simulink model "gm_Transformation_V12"  (R2018a)
settings: Solver=FixedStepDiscrete  StartTime=0.0  StopTime=10.0  RelTol=1e-3
InitFcn:
  | Ts_xadc = 0.1;
undefined symbols (not defined in the file or in its folder): T_25MHz, T_mech
libraries: hdlsllib x14, simulink x12, hdlmdlgenlib x5, simulink_need_slupdate x1
(part 3 of 4)

== matlab function gm_Transformation_V12/Trans_123_dq_fix_V3/dq_transformation ==
  data: a input; d output; b input; theta input; q output
% Author : Saeid Saeidi
% Modified: Sebastian Wendel
% EAL -TUM
% MATLAB Version : R2016a
function [d, q]= fcn(a,b, theta )
% Defining persistent variables
%In VHDL , persistent variables will appear as Signals
persistent i1
persistent i2
persistent i3
persistent i4
persistent i5
persistent i6
persistent i7
persistent i8
persistent i9
persistent i10
persistent i11
persistent i12
persistent i13
persistent i14
persistent i15
persistent i16
% %
persistent i1n
persistent i2n
persistent i3n
persistent i4n
persistent i5n
persistent i6n
persistent i7n
persistent i8n
persistent i9n
persistent i10n
persistent i11n
persistent i12n
persistent i13n
persistent i14n
persistent i15n
persistent i16n
% %
persistent a1
persistent a2
persistent a3
persistent a4
persistent a5
persistent a6
persistent a7
persistent a8
persistent a9
persistent a10
persistent a11
persistent a12
persistent a13
persistent a14
persistent a15
persistent a16
% %
persistent b1
persistent b2
persistent b3
persistent b4
persistent b5
persistent b6
persistent b7
persistent b8
persistent b9
persistent b10
persistent b11
persistent b12
persistent b13
persistent b14
persistent b15
persistent b16
% %
persistent beta1
persistent beta2
persistent beta3
persistent beta4
persistent beta5
persistent beta6
persistent beta7
persistent beta8
persistent beta9
persistent beta10
persistent beta11
persistent beta12
persistent beta13
persistent beta14
persistent beta15
% %
persistent a1n
persistent a2n
persistent a3n
persistent a4n
persistent a5n
persistent a6n
persistent a7n
persistent a8n
persistent a9n
persistent a10n
persistent a11n
persistent a12n
persistent a13n
persistent a14n
persistent a15n
persistent a16n
% %
persistent b1n
persistent b2n
persistent b3n
persistent b4n
persistent b5n
persistent b6n
persistent b7n
persistent b8n
persistent b9n
persistent b10n
persistent b11n
persistent b12n
persistent b13n
persistent b14n
persistent b15n
persistent b16n
% %
persistent beta1n
persistent beta2n
persistent beta3n
persistent beta4n
persistent beta5n
persistent beta6n
persistent beta7n
persistent beta8n
persistent beta9n
persistent beta10n
persistent beta11n
persistent beta12n
persistent beta13n
persistent beta14n
persistent beta15n
% %
% Initialization of Persistent Variables with the numeric type of the
% input variables "a" and "b"
% After generating VHDL this part will be located in the RESET
if isempty (a1)
a1 = fi (0, numerictype (a), hdlfimath );
a2 = fi (0, numerictype (a), hdlfimath );
a3 = fi (0, numerictype (a), hdlfimath );
a4 = fi (0, numerictype (a), hdlfimath );
a5 = fi (0, numerictype (a), hdlfimath );
a6 = fi (0, numerictype (a), hdlfimath );
a7 = fi (0, numerictype (a), hdlfimath );
a8 = fi (0, numerictype (a), hdlfimath );
a9 = fi (0, numerictype (a), hdlfimath );
a10 = fi (0, numerictype (a), hdlfimath );
a11 = fi (0, numerictype (a), hdlfimath );
a12 = fi (0, numerictype (a), hdlfimath );
a13 = fi (0, numerictype (a), hdlfimath );
a14 = fi (0, numerictype (a), hdlfimath );
a15 = fi (0, numerictype (a), hdlfimath );
a16 = fi (0, numerictype (a), hdlfimath );
% %
b1 = fi (0, numerictype (b), hdlfimath );
b2 = fi (0, numerictype (b), hdlfimath );
b3 = fi (0, numerictype (b), hdlfimath );
b4 = fi (0, numerictype (b), hdlfimath );
b5 = fi (0, numerictype (b), hdlfimath );
b6 = fi (0, numerictype (b), hdlfimath );
b7 = fi (0, numerictype (b), hdlfimath );
b8 = fi (0, numerictype (b), hdlfimath );
b9 = fi (0, numerictype (b), hdlfimath );
b10 = fi (0, numerictype (b), hdlfimath );
b11 = fi (0, numerictype (b), hdlfimath );
b12 = fi (0, numerictype (b), hdlfimath );
b13 = fi (0, numerictype (b), hdlfimath );
b14 = fi (0, numerictype (b), hdlfimath );
b15 = fi (0, numerictype (b), hdlfimath );
b16 = fi (0, numerictype (b), hdlfimath );
% %
beta1 = fi (0, numerictype ( theta ), hdlfimath );
beta2 = fi (0, numerictype ( theta ), hdlfimath );
beta3 = fi (0, numerictype ( theta ), hdlfimath );
beta4 = fi (0, numerictype ( theta ), hdlfimath );
beta5 = fi (0, numerictype ( theta ), hdlfimath );
beta6 = fi (0, numerictype ( theta ), hdlfimath );
beta7 = fi (0, numerictype ( theta ), hdlfimath );
beta8 = fi (0, numerictype ( theta ), hdlfimath );
beta9 = fi (0, numerictype ( theta ), hdlfimath );
beta10 = fi (0, numerictype ( theta ), hdlfimath );
beta11 = fi (0, numerictype ( theta ), hdlfimath );
beta12 = fi (0, numerictype ( theta ), hdlfimath );
beta13 = fi (0, numerictype ( theta ), hdlfimath );
beta14 = fi (0, numerictype ( theta ), hdlfimath );
beta15 = fi (0, numerictype ( theta ), hdlfimath );
% %
a1n = fi (0, numerictype (a), hdlfimath );
a2n = fi (0, numerictype (a), hdlfimath );
a3n = fi (0, numerictype (a), hdlfimath );
a4n = fi (0, numerictype (a), hdlfimath );
a5n = fi (0, numerictype (a), hdlfimath );
a6n = fi (0, numerictype (a), hdlfimath );
a7n = fi (0, numerictype (a), hdlfimath );
a8n = fi (0, numerictype (a), hdlfimath );
a9n = fi (0, numerictype (a), hdlfimath );
a10n = fi (0, numerictype (a), hdlfimath );
a11n = fi (0, numerictype (a), hdlfimath );
a12n = fi (0, numerictype (a), hdlfimath );
a13n = fi (0, numerictype (a), hdlfimath );
a14n = fi (0, numerictype (a), hdlfimath );
a15n = fi (0, numerictype (a), hdlfimath );
a16n = fi (0, numerictype (a), hdlfimath );
% %
b1n = fi (0, numerictype (b), hdlfimath );
b2n = fi (0, numerictype (b), hdlfimath );
b3n = fi (0, numerictype (b), hdlfimath );
b4n = fi (0, numerictype (b), hdlfimath );
b5n = fi (0, numerictype (b), hdlfimath );
b6n = fi (0, numerictype (b), hdlfimath );
b7n = fi (0, numerictype (b), hdlfimath );
b8n = fi (0, numerictype (b), hdlfimath );
b9n = fi (0, numerictype (b), hdlfimath );
b10n = fi (0, numerictype (b), hdlfimath );
b11n = fi (0, numerictype (b), hdlfimath );
b12n = fi (0, numerictype (b), hdlfimath );
b13n = fi (0, numerictype (b), hdlfimath );
b14n = fi (0, numerictype (b), hdlfimath );
b15n = fi (0, numerictype (b), hdlfimath );
b16n = fi (0, numerictype (b), hdlfimath );
% %
beta1n = fi (0, numerictype ( theta ), hdlfimath );
beta2n = fi (0, numerictype ( theta ), hdlfimath );
beta3n = fi (0, numerictype ( theta ), hdlfimath );
beta4n = fi (0, numerictype ( theta ), hdlfimath );
beta5n = fi (0, numerictype ( theta ), hdlfimath );
beta6n = fi (0, numerictype ( theta ), hdlfimath );
beta7n = fi (0, numerictype ( theta ), hdlfimath );
beta8n = fi (0, numerictype ( theta ), hdlfimath );
beta9n = fi (0, numerictype ( theta ), hdlfimath );
beta10n = fi (0, numerictype ( theta ), hdlfimath );
beta11n = fi (0, numerictype ( theta ), hdlfimath );
beta12n = fi (0, numerictype ( theta ), hdlfimath );
beta13n = fi (0, numerictype ( theta ), hdlfimath );
beta14n = fi (0, numerictype ( theta ), hdlfimath );
beta15n = fi (0, numerictype ( theta ), hdlfimath );
% %
i1n = ufi (0 ,1 ,0);
i2n = ufi (0 ,1 ,0);
i3n = ufi (0 ,1 ,0);
i4n = ufi (0 ,1 ,0);
i5n = ufi (0 ,1 ,0);
i6n = ufi (0 ,1 ,0);
i7n = ufi (0 ,1 ,0);
i8n = ufi (0 ,1 ,0);
i9n = ufi (0 ,1 ,0);
i10n = ufi (0 ,1 ,0);
i11n = ufi (0 ,1 ,0);
i12n = ufi (0 ,1 ,0);
i13n = ufi (0 ,1 ,0);
i14n = ufi (0 ,1 ,0);
i15n = ufi (0 ,1 ,0);
i16n = ufi (0 ,1 ,0);
% %
i1 = ufi (0 ,1 ,0);
i2 = ufi (0 ,1 ,0);
i3 = ufi (0 ,1 ,0);
i4 = ufi (0 ,1 ,0);
i5 = ufi (0 ,1 ,0);
i6 = ufi (0 ,1 ,0);
i7 = ufi (0 ,1 ,0);
i8 = ufi (0 ,1 ,0);
i9 = ufi (0 ,1 ,0);
i10 = ufi (0 ,1 ,0);
i11 = ufi (0 ,1 ,0);
i12 = ufi (0 ,1 ,0);
i13 = ufi (0 ,1 ,0);
i14 = ufi (0 ,1 ,0);
i15 = ufi (0 ,1 ,0);
i16 = ufi (0 ,1 ,0);
end
%-----------------------------------------------------------------------%

% Definition of Constant Values
p       = fi(pi , numerictype ( theta ), hdlfimath );
p2      = fi(pi /2, numerictype ( theta ), hdlfimath ); %1.570796
p2m     = fi(-pi /2, numerictype ( theta ), hdlfimath );
theta0  = fi(theta , numerictype ( theta ), hdlfimath );

% Determining section of the theta -> Check if theta is between -pi/2 and
% pi/2
% -- ------- # First pipeline stage
if( theta0 <= fi(p2m , numerictype ( theta ), hdlfimath ))
    beta1n = fi( theta0 + p, numerictype ( theta ), hdlfimath );
    i1n = ufi (0 ,1 ,0);
elseif ( theta0 >= fi(p2 , numerictype ( theta ), hdlfimath ))
    beta1n = fi( theta0 - p, numerictype ( theta ), hdlfimath );
    i1n = ufi (0 ,1 ,0);
else
    beta1n = theta0 ;
    i1n = ufi (1 ,1 ,0);
end
a1n = fi(a, numerictype (a), hdlfimath );
b1n = fi(b, numerictype (b), hdlfimath );

% -- ------- # Second pipeline stage 0.78539816339745 = pi/4
if( beta1 <fi (0, numerictype ( theta ), hdlfimath ))
    a2n = fi(a1 + b1 , numerictype (a), hdlfimath );
    b2n = fi(b1 - a1 , numerictype (b), hdlfimath );
    beta2n = fi( beta1 + fi (0.78539816339745 , numerictype ( theta ) ,...
    hdlfimath ), numerictype ( theta ), hdlfimath );
else
    a2n = fi(a1 - b1 , numerictype (a), hdlfimath );
    b2n = fi(b1 + a1 , numerictype (b), hdlfimath );
    beta2n = fi( beta1 - fi (0.78539816339745 , numerictype ( theta ) ,...
    hdlfimath ), numerictype ( theta ), hdlfimath );
end

% -- ------- # Third pipeline stage 0.46364760900081 = pi/8 ???
if(beta2 <fi (0, numerictype ( theta ), hdlfimath ))
    a3n = fi(a2 + bitsra (b2 ,1) , numerictype (b), hdlfimath );
    b3n = fi(b2 - bitsra (a2 ,1) , numerictype (a), hdlfimath );
    beta3n = fi( beta2 + fi (0.46364760900081 , numerictype ( theta ) ,...
    hdlfimath ), numerictype ( theta ), hdlfimath );
else
    a3n = fi(a2 - bitsra (b2 ,1) , numerictype (a), hdlfimath );
    b3n = fi(b2 + bitsra (a2 ,1) , numerictype (b), hdlfimath );
    beta3n = fi( beta2 - fi (0.46364760900081 , numerictype ( theta ) ,...
    hdlfimath ), numerictype ( theta ), hdlfimath );
end

% -- ------- # Fourth pipeline stage
if(beta3 <fi (0, numerictype ( theta ), hdlfimath ))
    a4n = fi(a3 + bitsra (b3 ,2) , numerictype (a), hdlfimath );
    b4n = fi(b3 - bitsra (a3 ,2) , numerictype (b), hdlfimath );
    beta4n = fi( beta3 + fi (0.24497866312686 , numerictype ( theta ) ,...
    hdlfimath ), numerictype ( theta ), hdlfimath );
else
    a4n = fi(a3 - bitsra (b3 ,2) , numerictype (a), hdlfimath );
    b4n = fi(b3 + bitsra (a3 ,2) , numerictype (b), hdlfimath );
    beta4n = fi( beta3 - fi (0.24497866312686 , numerictype ( theta ) ,...
    hdlfimath ), numerictype ( theta ), hdlfimath );
end

% -- ------- # Fifth pipeline stage
if(beta4 <fi (0, numerictype ( theta ), hdlfimath ))
    a5n = fi(a4 + bitsra (b4 ,3) , numerictype (a), hdlfimath );
    b5n = fi(b4 - bitsra (a4 ,3) , numerictype (b), hdlfimath );
    beta5n = fi( beta4 + fi (0.12435499454676 , numerictype ( theta ) ,...
    hdlfimath ), numerictype ( theta ), hdlfimath );
else
    a5n = fi(a4 - bitsra (b4 ,3) , numerictype (a), hdlfimath );
    b5n = fi(b4 + bitsra (a4 ,3) , numerictype (b), hdlfimath );
    beta5n = fi( beta4 - fi (0.12435499454676 , numerictype ( theta ) ,...
    hdlfimath ), numerictype ( theta ), hdlfimath );
end

% -- ------- # Sixth pipeline stage
if(beta5 <fi (0, numerictype ( theta ), hdlfimath ))
    a6n = fi(a5 + bitsra (b5 ,4) , numerictype (a), hdlfimath );
    b6n = fi(b5 - bitsra (a5 ,4) , numerictype (b), hdlfimath );
    beta6n = fi( beta5 + fi (0.06241880999596 , numerictype ( theta ) ,...
    hdlfimath ), numerictype ( theta ), hdlfimath );
else
    a6n = fi(a5 - bitsra (b5 ,4) , numerictype (a), hdlfimath );
    b6n = fi( b5 + bitsra (a5 ,4) , numerictype (b), hdlfimath );
    beta6n = fi( beta5 - fi (0.06241880999596 , numerictype ( theta ) ,...
    hdlfimath ), numerictype ( theta ), hdlfimath );
end

% -- ------- # Seventh pipeline stage
if(beta6 <fi (0, numerictype ( theta ), hdlfimath ))
    a7n = fi(a6 + bitsra (b6 ,5) , numerictype (a), hdlfimath );
    b7n = fi(b6 - bitsra (a6 ,5) , numerictype (b), hdlfimath );
    beta7n = fi( beta6 + fi (0.03123983343027 , numerictype ( theta ) ,...
    hdlfimath ), numerictype ( theta ), hdlfimath );
else
    a7n = fi(a6 - bitsra (b6 ,5) , numerictype (a), hdlfimath );
    b7n = fi(b6 + bitsra (a6 ,5) , numerictype (b), hdlfimath );
    beta7n = fi( beta6 - fi (0.03123983343027 , numerictype ( theta ) ,...
    hdlfimath ), numerictype ( theta ), hdlfimath );
end

% -- ------- # Eighth pipeline stage
if(beta7 <fi (0, numerictype ( theta ), hdlfimath ))
    a8n = fi(a7 + bitsra (b7 ,6) , numerictype (a), hdlfimath );
    b8n = fi(b7 - bitsra (a7 ,6) , numerictype (b), hdlfimath );
    beta8n = fi( beta7 + fi (0.01562372862048 , numerictype ( theta ) ,...
    hdlfimath ), numerictype ( theta ), hdlfimath );
else
    a8n = fi(a7 - bitsra (b7 ,6) , numerictype (a), hdlfimath );
    b8n = fi(b7 + bitsra (a7 ,6) , numerictype (b), hdlfimath );
    beta8n = fi( beta7 - fi (0.01562372862048 , numerictype ( theta ) ,...
    hdlfimath ), numerictype ( theta ), hdlfimath );
end

% -- ------- # Ninth pipeline stage
if(beta8 <fi (0, numerictype ( theta ), hdlfimath ))
    a9n = fi(a8 + bitsra (b8 ,7) , numerictype (a), hdlfimath );
    b9n = fi(b8 - bitsra (a8 ,7) , numerictype (b), hdlfimath );
    beta9n = fi( beta8 + fi( 0.00781234106010 , numerictype ( theta ) ,...
    hdlfimath ), numerictype ( theta ), hdlfimath );
else
    a9n = fi(a8 - bitsra (b8 ,7) , numerictype (a), hdlfimath );
    b9n = fi( b8 + bitsra (a8 ,7) , numerictype (b), hdlfimath );
    beta9n = fi( beta8 - fi( 0.00781234106010 , numerictype ( theta ) ,...
    hdlfimath ), numerictype ( theta ), hdlfimath );
end

% -- ------- # Tenth pipeline stage
if(beta9 <fi (0, numerictype ( theta ), hdlfimath ))
    a10n = fi(a9 + bitsra (b9 ,8) , numerictype (a), hdlfimath );
    b10n = fi(b9 - bitsra (a9 ,8) , numerictype (b), hdlfimath );
    beta10n = fi( beta9 + fi (0.00390623013197 , numerictype ( theta ) ,...
    hdlfimath ), numerictype ( theta ), hdlfimath );
else
    a10n = fi(a9 - bitsra (b9 ,8) , numerictype (a), hdlfimath );
    b10n = fi(b9 + bitsra (a9 ,8) , numerictype (b), hdlfimath );
    beta10n = fi( beta9 - fi (0.00390623013197 , numerictype ( theta ) ,...
    hdlfimath ), numerictype ( theta ), hdlfimath );
end

% -- ------- # Eleventh pipeline stage
if( beta10 <fi (0, numerictype ( theta ), hdlfimath ))
    a11n = fi(a10 + bitsra (b10 ,9) , numerictype (a), hdlfimath );
    b11n = fi(b10 - bitsra (a10 ,9) , numerictype (b), hdlfimath );
    beta11n = fi( beta10 + fi (0.00195312251648 , numerictype ( theta ) ,...
    hdlfimath ), numerictype ( theta ), hdlfimath );
else
    a11n = fi(a10 - bitsra (b10 ,9) , numerictype (a), hdlfimath );
    b11n = fi(b10 + bitsra (a10 ,9) , numerictype (b), hdlfimath );
    beta11n = fi( beta10 - fi (0.00195312251648 , numerictype ( theta ) ,...
    hdlfimath ), numerictype ( theta ), hdlfimath );
end

% -- ------- # Twelfth pipeline stage
if( beta11 <fi (0, numerictype ( theta ), hdlfimath ))
    a12n = fi( a11 + bitsra (b11 ,10) , numerictype (a), hdlfimath );
    b12n = fi(b11 - bitsra (a11 ,10) , numerictype (b), hdlfimath );
    beta12n = fi( beta11 + fi (0.00097656218956 , numerictype ( theta ) ,...
    hdlfimath ), numerictype ( theta ), hdlfimath );
else
    a12n = fi(a11 - bitsra (b11 ,10) , numerictype (a), hdlfimath );
    b12n = fi( b11 + bitsra (a11 ,10) , numerictype (b), hdlfimath );
    beta12n = fi( beta11 - fi (0.00097656218956 , numerictype ( theta ) ,...
    hdlfimath ), numerictype ( theta ), hdlfimath );
end

% -- ------- # Thirteenth pipeline stage
if( beta12 <fi (0, numerictype ( theta ), hdlfimath ))
    a13n = fi( a12 + bitsra (b12 ,11) , numerictype (a), hdlfimath );
    b13n = fi(b12 - bitsra (a12 ,11) , numerictype (b), hdlfimath );
    beta13n = fi( beta12 + fi (0.00048828121119 ,numerictype ( theta ) ,...
    hdlfimath ), numerictype ( theta ), hdlfimath );
else
    a13n = fi(a12 - bitsra (b12 ,11) , numerictype (a), hdlfimath );
    b13n = fi( b12 + bitsra (a12 ,11) , numerictype (b), hdlfimath );
    beta13n = fi( beta12 - fi (0.00048828121119 ,numerictype ( theta ) ,...
    hdlfimath ), numerictype ( theta ), hdlfimath );
end

% -- ------- # Fourteenth pipeline stage
if( beta13 <fi (0, numerictype ( theta ), hdlfimath ))
    a14n = fi( a13 + bitsra (b13 ,12) , numerictype (a), hdlfimath );
    b14n = fi(b13 - bitsra (a13 ,12) , numerictype (b), hdlfimath );
    beta14n = fi( beta13 + fi( 0.00024414062015 , numerictype ( theta ) ,...
    hdlfimath ), numerictype ( theta ), hdlfimath );
else
    a14n = fi(a13 - bitsra (b13 ,12) , numerictype (a), hdlfimath );
    b14n = fi( b13 + bitsra (a13 ,12) , numerictype (b), hdlfimath );
    beta14n = fi( beta11 - fi( 0.00024414062015 , numerictype ( theta ) ,...
    hdlfimath ), numerictype ( theta ), hdlfimath );
end

% -- ------- # Fifteenth pipeline stage
if( beta14 <fi (0, numerictype ( theta ), hdlfimath ))
    a15n = fi( a14 + bitsra (b14 ,13) , numerictype (a), hdlfimath );
    b15n = fi(b14 - bitsra (a14 ,13) , numerictype (b), hdlfimath );
    beta15n = fi( beta14 + fi (0.00012207031189 , numerictype ( theta ) ,...
    hdlfimath ), numerictype ( theta ), hdlfimath );
else
    a15n = fi(a14 - bitsra (b14 ,13) , numerictype (a), hdlfimath );
    b15n = fi( b14 + bitsra (a14 ,13) , numerictype (b), hdlfimath );
    beta15n = fi( beta14 - fi (0.00012207031189 , numerictype ( theta ) ,...
    hdlfimath ), numerictype ( theta ), hdlfimath );
end

% -- ------- # Sixteenth pipeline stage
a16n = fi(a15 * sfi ( 0.60725293538591 ,18 ,17) , numerictype (a), hdlfimath );
b16n = fi(b15 * sfi ( 0.60725293538591 ,18 ,17) , numerictype (b), hdlfimath );

% Output Update of Registers
i2n = i1;
i3n = i2;
i4n = i3;
i5n = i4;
i6n = i5;
i7n = i6;
i8n = i7;
i9n = i8;
i10n = i9;
i11n = i10 ;
i12n = i11 ;
i13n = i12 ;
i14n = i13 ;
i15n = i14 ;
i16n = i15 ;
% %
a1 = a1n;
a2 = a2n;
a3 = a3n;
a4 = a4n;
a5 = a5n;
a6 = a6n;
a7 = a7n;
a8 = a8n;
a9 = a9n;
a10 = a10n ;
a11 = a11n ;
a12 = a12n ;
a13 = a13n ;
a14 = a14n ;
a15 = a15n ;
a16 = a16n ;
% %
b1 = b1n;
b2 = b2n;
b3 = b3n;
b4 = b4n;
b5 = b5n;
b6 = b6n;
b7 = b7n;
b8 = b8n;
b9 = b9n;
b10 = b10n ;

b11 = b11n ;
b12 = b12n ;
b13 = b13n ;
b14 = b14n ;
b15 = b15n ;
b16 = b16n ;
% %
beta1 = beta1n ;
beta2 = beta2n ;
beta3 = beta3n ;
beta4 = beta4n ;
beta5 = beta5n ;
beta6 = beta6n ;
beta7 = beta7n ;
beta8 = beta8n ;
beta9 = beta9n ;
beta10 = beta10n ;
beta11 = beta11n ;
beta12 = beta12n ;
beta13 = beta13n ;
beta14 = beta14n ;
beta15 = beta15n ;
% %
i1 = i1n;
i2 = i2n;
i3 = i3n;
i4 = i4n;
i5 = i5n;
i6 = i6n;
i7 = i7n;
i8 = i8n;
i9 = i9n;
i10 = i10n ;
i11 = i11n ;
i12 = i12n ;
i13 = i13n ;
i14 = i14n ;
i15 = i15n ;
i16 = i16n ;
% %
% Generating output
if( i16 == ufi (0 ,1 ,0))
d = -a16;
q = -b16;
else
d = a16;
q = b16;
end

== matlab function gm_Transformation_V12/DUT_V5/xadc_ctrl ==
  data: den_o output; drdy_i input; daddr_o output; do_i input; val_o output
function [den_o, daddr_o, val_o] = xadc_ctrl(drdy_i, do_i)
%#codegen

%% Constants and defines
% Fixed point data types
FM = hdlfimath;
NT_ADDR = numerictype(false,7,0); % Address
NT_VAL = numerictype(false,16,0); % Value
NT_STATE = numerictype(false,2,0); % State

% The state machine will loop over the defined addresses
% reading out each value
% See Xilinx ug480 for more information
ADDR_SEQ = fi([0 1 3 16 24], ... % Value addresses
               NT_ADDR,FM);

NUM_VALS = numel(ADDR_SEQ); % Number of values to read

% Define the index data type based on the number of values
NT_ADDR_IDX = numerictype(false,ceil(log2(NUM_VALS))+1,0); % index

% State machine defines
STATE_IDLE = fi(0,NT_STATE,FM);           
STATE_ADDR = fi(1,NT_STATE,FM);
STATE_EN = fi(2,NT_STATE,FM);
STATE_WAIT = fi(3,NT_STATE,FM);
           
% Declare registers
persistent state val addr den addr_idx;

% Set reset values
if isempty(state)
    state = STATE_IDLE;
    val = fi(zeros(NUM_VALS,1),NT_VAL,FM);
    addr = fi(0,NT_ADDR,FM);
    den = false;
    addr_idx = fi(0,NT_ADDR_IDX,FM);
end

%% Drive the outputs
daddr_o = addr;
den_o = den;
val_o = val;

%% Control the state
switch (state)
    case STATE_IDLE
        % IDLE state, increment the index
        if (addr_idx == NUM_VALS)
            addr_idx(:) = 1;
        else
            addr_idx(:) = addr_idx + 1;
        end
        state(:) = STATE_ADDR;
    case STATE_ADDR
        % ADDR state, write out the address
        addr(:) = ADDR_SEQ(addr_idx);
        den(:) = false;
        state(:) = STATE_EN;
    case STATE_EN
        % EN state, drive the enable high
        state(:) = STATE_WAIT;
        den(:) = true;
    case STATE_WAIT
        % WAIT state, wait for drdy
        if (drdy_i)
            val(addr_idx) = do_i;
            state(:) = STATE_IDLE;
        end
        den(:) = false;
end

== matlab function gm_Transformation_V12/Trans_123_dq_fix_V11/dq_transformation ==
  data: a input; d output; b input; theta input; q output
% Author : Saeid Saeidi
% Modified: Sebastian Wendel
% EAL -TUM
% MATLAB Version : R2016a
function [d, q]= fcn(a,b, theta )
% Defining persistent variables
%In VHDL , persistent variables will appear as Signals
persistent i1
persistent i2
persistent i3
persistent i4
persistent i5
persistent i6
persistent i7
persistent i8
persistent i9
persistent i10
persistent i11
persistent i12
persistent i13
persistent i14
persistent i15
persistent i16
% %
persistent i1n
persistent i2n
persistent i3n
persistent i4n
persistent i5n
persistent i6n
persistent i7n
persistent i8n
persistent i9n
persistent i10n
persistent i11n
persistent i12n
persistent i13n
persistent i14n
persistent i15n
persistent i16n
% %
persistent a1
persistent a2
persistent a3
persistent a4
persistent a5
persistent a6
persistent a7
persistent a8
persistent a9
persistent a10
persistent a11
persistent a12
persistent a13
persistent a14
persistent a15
persistent a16
% %
persistent b1
persistent b2
persistent b3
persistent b4
persistent b5
persistent b6
persistent b7
persistent b8
persistent b9
persistent b10
persistent b11
persistent b12
persistent b13
persistent b14
persistent b15
persistent b16
% %
persistent beta1
persistent beta2
persistent beta3
persistent beta4
persistent beta5
persistent beta6
persistent beta7
persistent beta8
persistent beta9
persistent beta10
persistent beta11
persistent beta12
persistent beta13
persistent beta14
persistent beta15
% %
persistent a1n
persistent a2n
persistent a3n
persistent a4n
persistent a5n
persistent a6n
persistent a7n
persistent a8n
persistent a9n
persistent a10n
persistent a11n
persistent a12n
persistent a13n
persistent a14n
persistent a15n
persistent a16n
% %
persistent b1n
persistent b2n
persistent b3n
persistent b4n
persistent b5n
persistent b6n
persistent b7n
persistent b8n
persistent b9n
persistent b10n
persistent b11n
persistent b12n
persistent b13n
persistent b14n
persistent b15n
persistent b16n
% %
persistent beta1n
persistent beta2n
persistent beta3n
persistent beta4n
persistent beta5n
persistent beta6n
persistent beta7n
persistent beta8n
persistent beta9n
persistent beta10n
persistent beta11n
persistent beta12n
persistent beta13n
persistent beta14n
persistent beta15n
% %
% Initialization of Persistent Variables with the numeric type of the
% input variables "a" and "b"
% After generating VHDL this part will be located in the RESET
if isempty (a1)
a1 = fi (0, numerictype (a), hdlfimath );
a2 = fi (0, numerictype (a), hdlfimath );
a3 = fi (0, numerictype (a), hdlfimath );
a4 = fi (0, numerictype (a), hdlfimath );
a5 = fi (0, numerictype (a), hdlfimath );
a6 = fi (0, numerictype (a), hdlfimath );
a7 = fi (0, numerictype (a), hdlfimath );
a8 = fi (0, numerictype (a), hdlfimath );
a9 = fi (0, numerictype (a), hdlfimath );
a10 = fi (0, numerictype (a), hdlfimath );
a11 = fi (0, numerictype (a), hdlfimath );
a12 = fi (0, numerictype (a), hdlfimath );
a13 = fi (0, numerictype (a), hdlfimath );
a14 = fi (0, numerictype (a), hdlfimath );
a15 = fi (0, numerictype (a), hdlfimath );
a16 = fi (0, numerictype (a), hdlfimath );
% %
b1 = fi (0, numerictype (b), hdlfimath );
b2 = fi (0, numerictype (b), hdlfimath );
b3 = fi (0, numerictype (b), hdlfimath );
b4 = fi (0, numerictype (b), hdlfimath );
b5 = fi (0, numerictype (b), hdlfimath );
b6 = fi (0, numerictype (b), hdlfimath );
b7 = fi (0, numerictype (b), hdlfimath );
b8 = fi (0, numerictype (b), hdlfimath );
b9 = fi (0, numerictype (b), hdlfimath );
b10 = fi (0, numerictype (b), hdlfimath );
b11 = fi (0, numerictype (b), hdlfimath );
b12 = fi (0, numerictype (b), hdlfimath );
b13 = fi (0, numerictype (b), hdlfimath );
b14 = fi (0, numerictype (b), hdlfimath );
b15 = fi (0, numerictype (b), hdlfimath );
b16 = fi (0, numerictype (b), hdlfimath );
% %
beta1 = fi (0, numerictype ( theta ), hdlfimath );
beta2 = fi (0, numerictype ( theta ), hdlfimath );
beta3 = fi (0, numerictype ( theta ), hdlfimath );
beta4 = fi (0, numerictype ( theta ), hdlfimath );
beta5 = fi (0, numerictype ( theta ), hdlfimath );
beta6 = fi (0, numerictype ( theta ), hdlfimath );
beta7 = fi (0, numerictype ( theta ), hdlfimath );
beta8 = fi (0, numerictype ( theta ), hdlfimath );
beta9 = fi (0, numerictype ( theta ), hdlfimath );
beta10 = fi (0, numerictype ( theta ), hdlfimath );
beta11 = fi (0, numerictype ( theta ), hdlfimath );
beta12 = fi (0, numerictype ( theta ), hdlfimath );
beta13 = fi (0, numerictype ( theta ), hdlfimath );
beta14 = fi (0, numerictype ( theta ), hdlfimath );
beta15 = fi (0, numerictype ( theta ), hdlfimath );
% %
a1n = fi (0, numerictype (a), hdlfimath );
a2n = fi (0, numerictype (a), hdlfimath );
a3n = fi (0, numerictype (a), hdlfimath );
a4n = fi (0, numerictype (a), hdlfimath );
a5n = fi (0, numerictype (a), hdlfimath );
a6n = fi (0, numerictype (a), hdlfimath );
a7n = fi (0, numerictype (a), hdlfimath );
a8n = fi (0, numerictype (a), hdlfimath );
a9n = fi (0, numerictype (a), hdlfimath );
a10n = fi (0, numerictype (a), hdlfimath );
a11n = fi (0, numerictype (a), hdlfimath );
a12n = fi (0, numerictype (a), hdlfimath );
a13n = fi (0, numerictype (a), hdlfimath );
a14n = fi (0, numerictype (a), hdlfimath );
a15n = fi (0, numerictype (a), hdlfimath );
a16n = fi (0, numerictype (a), hdlfimath );
% %
b1n = fi (0, numerictype (b), hdlfimath );
b2n = fi (0, numerictype (b), hdlfimath );
b3n = fi (0, numerictype (b), hdlfimath );
b4n = fi (0, numerictype (b), hdlfimath );
b5n = fi (0, numerictype (b), hdlfimath );
b6n = fi (0, numerictype (b), hdlfimath );
b7n = fi (0, numerictype (b), hdlfimath );
b8n = fi (0, numerictype (b), hdlfimath );
b9n = fi (0, numerictype (b), hdlfimath );
b10n = fi (0, numerictype (b), hdlfimath );
b11n = fi (0, numerictype (b), hdlfimath );
b12n = fi (0, numerictype (b), hdlfimath );
b13n = fi (0, numerictype (b), hdlfimath );
b14n = fi (0, numerictype (b), hdlfimath );
b15n = fi (0, numerictype (b), hdlfimath );
b16n = fi (0, numerictype (b), hdlfimath );
% %
beta1n = fi (0, numerictype ( theta ), hdlfimath );
beta2n = fi (0, numerictype ( theta ), hdlfimath );
beta3n = fi (0, numerictype ( theta ), hdlfimath );
beta4n = fi (0, numerictype ( theta ), hdlfimath );
beta5n = fi (0, numerictype ( theta ), hdlfimath );
beta6n = fi (0, numerictype ( theta ), hdlfimath );
beta7n = fi (0, numerictype ( theta ), hdlfimath );
beta8n = fi (0, numerictype ( theta ), hdlfimath );
beta9n = fi (0, numerictype ( theta ), hdlfimath );
beta10n = fi (0, numerictype ( theta ), hdlfimath );
beta11n = fi (0, numerictype ( theta ), hdlfimath );
beta12n = fi (0, numerictype ( theta ), hdlfimath );
beta13n = fi (0, numerictype ( theta ), hdlfimath );
beta14n = fi (0, numerictype ( theta ), hdlfimath );
beta15n = fi (0, numerictype ( theta ), hdlfimath );
% %
i1n = ufi (0 ,1 ,0);
i2n = ufi (0 ,1 ,0);
i3n = ufi (0 ,1 ,0);
i4n = ufi (0 ,1 ,0);
i5n = ufi (0 ,1 ,0);
i6n = ufi (0 ,1 ,0);
i7n = ufi (0 ,1 ,0);
i8n = ufi (0 ,1 ,0);
i9n = ufi (0 ,1 ,0);
i10n = ufi (0 ,1 ,0);
i11n = ufi (0 ,1 ,0);
i12n = ufi (0 ,1 ,0);
i13n = ufi (0 ,1 ,0);
i14n = ufi (0 ,1 ,0);
i15n = ufi (0 ,1 ,0);
i16n = ufi (0 ,1 ,0);
% %
i1 = ufi (0 ,1 ,0);
i2 = ufi (0 ,1 ,0);
i3 = ufi (0 ,1 ,0);
i4 = ufi (0 ,1 ,0);
i5 = ufi (0 ,1 ,0);
i6 = ufi (0 ,1 ,0);
i7 = ufi (0 ,1 ,0);
i8 = ufi (0 ,1 ,0);
i9 = ufi (0 ,1 ,0);
i10 = ufi (0 ,1 ,0);
i11 = ufi (0 ,1 ,0);
i12 = ufi (0 ,1 ,0);
i13 = ufi (0 ,1 ,0);
i14 = ufi (0 ,1 ,0);
i15 = ufi (0 ,1 ,0);
i16 = ufi (0 ,1 ,0);
end
%-----------------------------------------------------------------------%

% Definition of Constant Values
p       = fi(pi , numerictype ( theta ), hdlfimath );
p2      = fi(pi /2, numerictype ( theta ), hdlfimath ); %1.570796
p2m     = fi(-pi /2, numerictype ( theta ), hdlfimath );
theta0  = fi(theta , numerictype ( theta ), hdlfimath );

% Determining section of the theta -> Check if theta is between -pi/2 and
% pi/2
% -- ------- # First pipeline stage
if( theta0 <= fi(p2m , numerictype ( theta ), hdlfimath ))
    beta1n = fi( theta0 + p, numerictype ( theta ), hdlfimath );
    i1n = ufi (0 ,1 ,0);
elseif ( theta0 >= fi(p2 , numerictype ( theta ), hdlfimath ))
    beta1n = fi( theta0 - p, numerictype ( theta ), hdlfimath );
    i1n = ufi (0 ,1 ,0);
else
    beta1n = theta0 ;
    i1n = ufi (1 ,1 ,0);
end
a1n = fi(a, numerictype (a), hdlfimath );
b1n = fi(b, numerictype (b), hdlfimath );

% -- ------- # Second pipeline stage 0.78539816339745 = pi/4
if( beta1 <fi (0, numerictype ( theta ), hdlfimath ))
    a2n = fi(a1 + b1 , numerictype (a), hdlfimath );
    b2n = fi(b1 - a1 , numerictype (b), hdlfimath );
    beta2n = fi( beta1 + fi (0.78539816339745 , numerictype ( theta ) ,...
    hdlfimath ), numerictype ( theta ), hdlfimath );
else
    a2n = fi(a1 - b1 , numerictype (a), hdlfimath );
    b2n = fi(b1 + a1 , numerictype (b), hdlfimath );
    beta2n = fi( beta1 - fi (0.78539816339745 , numerictype ( theta ) ,...
    hdlfimath ), numerictype ( theta ), hdlfimath );
end

% -- ------- # Third pipeline stage 0.46364760900081 = pi/8 ???
if(beta2 <fi (0, numerictype ( theta ), hdlfimath ))
    a3n = fi(a2 + bitsra (b2 ,1) , numerictype (b), hdlfimath );
    b3n = fi(b2 - bitsra (a2 ,1) , numerictype (a), hdlfimath );
    beta3n = fi( beta2 + fi (0.46364760900081 , numerictype ( theta ) ,...
    hdlfimath ), numerictype ( theta ), hdlfimath );
else
    a3n = fi(a2 - bitsra (b2 ,1) , numerictype (a), hdlfimath );
    b3n = fi(b2 + bitsra (a2 ,1) , numerictype (b), hdlfimath );
    beta3n = fi( beta2 - fi (0.46364760900081 , numerictype ( theta ) ,...
    hdlfimath ), numerictype ( theta ), hdlfimath );
end

% -- ------- # Fourth pipeline stage
if(beta3 <fi (0, numerictype ( theta ), hdlfimath ))
    a4n = fi(a3 + bitsra (b3 ,2) , numerictype (a), hdlfimath );
    b4n = fi(b3 - bitsra (a3 ,2) , numerictype (b), hdlfimath );
    beta4n = fi( beta3 + fi (0.24497866312686 , numerictype ( theta ) ,...
    hdlfimath ), numerictype ( theta ), hdlfimath );
else
    a4n = fi(a3 - bitsra (b3 ,2) , numerictype (a), hdlfimath );
    b4n = fi(b3 + bitsra (a3 ,2) , numerictype (b), hdlfimath );
    beta4n = fi( beta3 - fi (0.24497866312686 , numerictype ( theta ) ,...
    hdlfimath ), numerictype ( theta ), hdlfimath );
end

% -- ------- # Fifth pipeline stage
if(beta4 <fi (0, numerictype ( theta ), hdlfimath ))
    a5n = fi(a4 + bitsra (b4 ,3) , numerictype (a), hdlfimath );
    b5n = fi(b4 - bitsra (a4 ,3) , numerictype (b), hdlfimath );
    beta5n = fi( beta4 + fi (0.12435499454676 , numerictype ( theta ) ,...
    hdlfimath ), numerictype ( theta ), hdlfimath );
else
    a5n = fi(a4 - bitsra (b4 ,3) , numerictype (a), hdlfimath );
    b5n = fi(b4 + bitsra (a4 ,3) , numerictype (b), hdlfimath );
    beta5n = fi( beta4 - fi (0.12435499454676 , numerictype ( theta ) ,...
    hdlfimath ), numerictype ( theta ), hdlfimath );
end

% -- ------- # Sixth pipeline stage
if(beta5 <fi (0, numerictype ( theta ), hdlfimath ))
    a6n = fi(a5 + bitsra (b5 ,4) , numerictype (a), hdlfimath );
    b6n = fi(b5 - bitsra (a5 ,4) , numerictype (b), hdlfimath );
    beta6n = fi( beta5 + fi (0.06241880999596 , numerictype ( theta ) ,...
    hdlfimath ), numerictype ( theta ), hdlfimath );
else
    a6n = fi(a5 - bitsra (b5 ,4) , numerictype (a), hdlfimath );
    b6n = fi( b5 + bitsra (a5 ,4) , numerictype (b), hdlfimath );
    beta6n = fi( beta5 - fi (0.06241880999596 , numerictype ( theta ) ,...
    hdlfimath ), numerictype ( theta ), hdlfimath );
end

% -- ------- # Seventh pipeline stage
if(beta6 <fi (0, numerictype ( theta ), hdlfimath ))
    a7n = fi(a6 + bitsra (b6 ,5) , numerictype (a), hdlfimath );
    b7n = fi(b6 - bitsra (a6 ,5) , numerictype (b), hdlfimath );
    beta7n = fi( beta6 + fi (0.03123983343027 , numerictype ( theta ) ,...
    hdlfimath ), numerictype ( theta ), hdlfimath );
else
    a7n = fi(a6 - bitsra (b6 ,5) , numerictype (a), hdlfimath );
    b7n = fi(b6 + bitsra (a6 ,5) , numerictype (b), hdlfimath );
    beta7n = fi( beta6 - fi (0.03123983343027 , numerictype ( theta ) ,...
    hdlfimath ), numerictype ( theta ), hdlfimath );
end

% -- ------- # Eighth pipeline stage
if(beta7 <fi (0, numerictype ( theta ), hdlfimath ))
    a8n = fi(a7 + bitsra (b7 ,6) , numerictype (a), hdlfimath );
    b8n = fi(b7 - bitsra (a7 ,6) , numerictype (b), hdlfimath );
    beta8n = fi( beta7 + fi (0.01562372862048 , numerictype ( theta ) ,...
    hdlfimath ), numerictype ( theta ), hdlfimath );
else
    a8n = fi(a7 - bitsra (b7 ,6) , numerictype (a), hdlfimath );
    b8n = fi(b7 + bitsra (a7 ,6) , numerictype (b), hdlfimath );
    beta8n = fi( beta7 - fi (0.01562372862048 , numerictype ( theta ) ,...
    hdlfimath ), numerictype ( theta ), hdlfimath );
end

% -- ------- # Ninth pipeline stage
if(beta8 <fi (0, numerictype ( theta ), hdlfimath ))
    a9n = fi(a8 + bitsra (b8 ,7) , numerictype (a), hdlfimath );
    b9n = fi(b8 - bitsra (a8 ,7) , numerictype (b), hdlfimath );
    beta9n = fi( beta8 + fi( 0.00781234106010 , numerictype ( theta ) ,...
    hdlfimath ), numerictype ( theta ), hdlfimath );
else
    a9n = fi(a8 - bitsra (b8 ,7) , numerictype (a), hdlfimath );
    b9n = fi( b8 + bitsra (a8 ,7) , numerictype (b), hdlfimath );
    beta9n = fi( beta8 - fi( 0.00781234106010 , numerictype ( theta ) ,...
    hdlfimath ), numerictype ( theta ), hdlfimath );
end

% -- ------- # Tenth pipeline stage
if(beta9 <fi (0, numerictype ( theta ), hdlfimath ))
    a10n = fi(a9 + bitsra (b9 ,8) , numerictype (a), hdlfimath );
    b10n = fi(b9 - bitsra (a9 ,8) , numerictype (b), hdlfimath );
    beta10n = fi( beta9 + fi (0.00390623013197 , numerictype ( theta ) ,...
    hdlfimath ), numerictype ( theta ), hdlfimath );
else
    a10n = fi(a9 - bitsra (b9 ,8) , numerictype (a), hdlfimath );
    b10n = fi(b9 + bitsra (a9 ,8) , numerictype (b), hdlfimath );
    beta10n = fi( beta9 - fi (0.00390623013197 , numerictype ( theta ) ,...
    hdlfimath ), numerictype ( theta ), hdlfimath );
end

% -- ------- # Eleventh pipeline stage
if( beta10 <fi (0, numerictype ( theta ), hdlfimath ))
    a11n = fi(a10 + bitsra (b10 ,9) , numerictype (a), hdlfimath );
    b11n = fi(b10 - bitsra (a10 ,9) , numerictype (b), hdlfimath );
    beta11n = fi( beta10 + fi (0.00195312251648 , numerictype ( theta ) ,...
    hdlfimath ), numerictype ( theta ), hdlfimath );
else
    a11n = fi(a10 - bitsra (b10 ,9) , numerictype (a), hdlfimath );
    b11n = fi(b10 + bitsra (a10 ,9) , numerictype (b), hdlfimath );
    beta11n = fi( beta10 - fi (0.00195312251648 , numerictype ( theta ) ,...
    hdlfimath ), numerictype ( theta ), hdlfimath );
end

% -- ------- # Twelfth pipeline stage
if( beta11 <fi (0, numerictype ( theta ), hdlfimath ))
    a12n = fi( a11 + bitsra (b11 ,10) , numerictype (a), hdlfimath );
    b12n = fi(b11 - bitsra (a11 ,10) , numerictype (b), hdlfimath );
    beta12n = fi( beta11 + fi (0.00097656218956 , numerictype ( theta ) ,...
    hdlfimath ), numerictype ( theta ), hdlfimath );
else
    a12n = fi(a11 - bitsra (b11 ,10) , numerictype (a), hdlfimath );
    b12n = fi( b11 + bitsra (a11 ,10) , numerictype (b), hdlfimath );
    beta12n = fi( beta11 - fi (0.00097656218956 , numerictype ( theta ) ,...
    hdlfimath ), numerictype ( theta ), hdlfimath );
end

% -- ------- # Thirteenth pipeline stage
if( beta12 <fi (0, numerictype ( theta ), hdlfimath ))
    a13n = fi( a12 + bitsra (b12 ,11) , numerictype (a), hdlfimath );
    b13n = fi(b12 - bitsra (a12 ,11) , numerictype (b), hdlfimath );
    beta13n = fi( beta12 + fi (0.00048828121119 ,numerictype ( theta ) ,...
    hdlfimath ), numerictype ( theta ), hdlfimath );
else
    a13n = fi(a12 - bitsra (b12 ,11) , numerictype (a), hdlfimath );
    b13n = fi( b12 + bitsra (a12 ,11) , numerictype (b), hdlfimath );
    beta13n = fi( beta12 - fi (0.00048828121119 ,numerictype ( theta ) ,...
    hdlfimath ), numerictype ( theta ), hdlfimath );
end

% -- ------- # Fourteenth pipeline stage
if( beta13 <fi (0, numerictype ( theta ), hdlfimath ))
    a14n = fi( a13 + bitsra (b13 ,12) , numerictype (a), hdlfimath );
    b14n = fi(b13 - bitsra (a13 ,12) , numerictype (b), hdlfimath );
    beta14n = fi( beta13 + fi( 0.00024414062015 , numerictype ( theta ) ,...
    hdlfimath ), numerictype ( theta ), hdlfimath );
else
    a14n = fi(a13 - bitsra (b13 ,12) , numerictype (a), hdlfimath );
    b14n = fi( b13 + bitsra (a13 ,12) , numerictype (b), hdlfimath );
    beta14n = fi( beta11 - fi( 0.00024414062015 , numerictype ( theta ) ,...
    hdlfimath ), numerictype ( theta ), hdlfimath );
end

% -- ------- # Fifteenth pipeline stage
if( beta14 <fi (0, numerictype ( theta ), hdlfimath ))
    a15n = fi( a14 + bitsra (b14 ,13) , numerictype (a), hdlfimath );
    b15n = fi(b14 - bitsra (a14 ,13) , numerictype (b), hdlfimath );
    beta15n = fi( beta14 + fi (0.00012207031189 , numerictype ( theta ) ,...
    hdlfimath ), numerictype ( theta ), hdlfimath );
else
    a15n = fi(a14 - bitsra (b14 ,13) , numerictype (a), hdlfimath );
    b15n = fi( b14 + bitsra (a14 ,13) , numerictype (b), hdlfimath );
    beta15n = fi( beta14 - fi (0.00012207031189 , numerictype ( theta ) ,...
    hdlfimath ), numerictype ( theta ), hdlfimath );
end

% -- ------- # Sixteenth pipeline stage
a16n = fi(a15 * sfi ( 0.60725293538591 ,18 ,17) , numerictype (a), hdlfimath );
b16n = fi(b15 * sfi ( 0.60725293538591 ,18 ,17) , numerictype (b), hdlfimath );

% Output Update of Registers
i2n = i1;
i3n = i2;
i4n = i3;
i5n = i4;
i6n = i5;
i7n = i6;
i8n = i7;
i9n = i8;
i10n = i9;
i11n = i10 ;
i12n = i11 ;
i13n = i12 ;
i14n = i13 ;
i15n = i14 ;
i16n = i15 ;
% %
a1 = a1n;
a2 = a2n;
a3 = a3n;
a4 = a4n;
a5 = a5n;
a6 = a6n;
a7 = a7n;
a8 = a8n;
a9 = a9n;
a10 = a10n ;
a11 = a11n ;
a12 = a12n ;
a13 = a13n ;
a14 = a14n ;
a15 = a15n ;
a16 = a16n ;
% %
b1 = b1n;
b2 = b2n;
b3 = b3n;
b4 = b4n;
b5 = b5n;
b6 = b6n;
b7 = b7n;
b8 = b8n;
b9 = b9n;
b10 = b10n ;

b11 = b11n ;
b12 = b12n ;
b13 = b13n ;
b14 = b14n ;
b15 = b15n ;
b16 = b16n ;
% %
beta1 = beta1n ;
beta2 = beta2n ;
beta3 = beta3n ;
beta4 = beta4n ;
beta5 = beta5n ;
beta6 = beta6n ;
beta7 = beta7n ;
beta8 = beta8n ;
beta9 = beta9n ;
beta10 = beta10n ;
beta11 = beta11n ;
beta12 = beta12n ;
beta13 = beta13n ;
beta14 = beta14n ;
beta15 = beta15n ;
% %
i1 = i1n;
i2 = i2n;
i3 = i3n;
i4 = i4n;
i5 = i5n;
i6 = i6n;
i7 = i7n;
i8 = i8n;
i9 = i9n;
i10 = i10n ;
i11 = i11n ;
i12 = i12n ;
i13 = i13n ;
i14 = i14n ;
i15 = i15n ;
i16 = i16n ;
% %
% Generating output
if( i16 == ufi (0 ,1 ,0))
d = -a16;
q = -b16;
else
d = a16;
q = b16;
end
